simulink model "quadRotorController"  (R2016a)
settings: Solver=VariableStepAuto  StartTime=0.0  StopTime=100  RelTol=1e-3
libraries: simulink x1
settings Model: Creator=Nariman  LastModifiedBy=Nariman

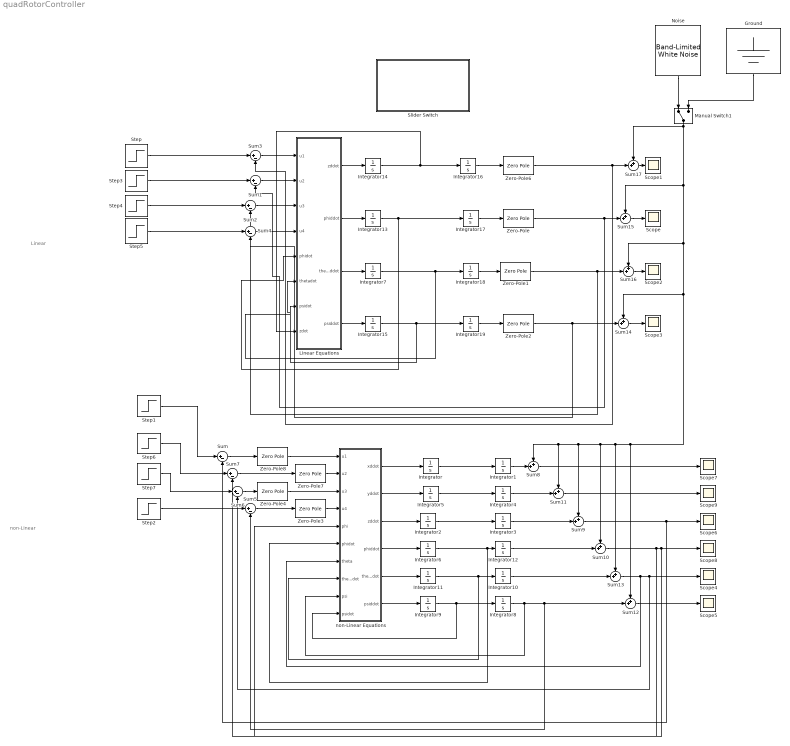
== system quadRotorController ==
  note: non-Linear
  note: Linear
  Ground : Ground
  Integrator{,1..19} (20 alike) : Integrator
  Linear Equations : MATLAB Function  TreatAsAtomicUnit=on
  Manual Switch1 : ManualSwitch
  Noise : simulink/Sources/Band-Limited White Noise  Cov=0.0000000001  Ts=0.1  seed=[23341]
  Scope{,1..9} (10 alike) : Scope
  Slider Switch : Subsystem  DialogController=hmiCreateDDGDialog  IsWebBlock=on  mask(MWDashboardBlock){webBlockId=d59a5245-7345-4851-88b2-e95f32656578, webBlockType=sliderswitch, ShowInLibBrowser=on, ShowInitialText=on, HMISrcModelName=model}
      mask prompts: webBlockId "WebBlock Id"; webBlockType "WebBlock Type"; HMISrcModelName "Source Model"
      mask Help: helpview([docroot '/mapfiles/simulink.map'], 'hmi_slider_switch')
      mask Display:
      | if strcmp(get_param(bdroot(gcb),'BlockDiagramType'), 'library')
      |     image([(matlabroot) '/toolbox/simulink/hmi/icons/SliderSwitch.png']);
      | end
  Step{,3..7} (6 alike) : Step  After=0.01  SampleTime=0
  Step1 : Step  After=90  SampleTime=0
  Step2 : Step  After=90  SampleTime=0
  Sum{,1..7} (8 alike) : Sum  Inputs=|+-
  Sum{8..17} (10 alike) : Sum  Inputs=++|
  Zero-Pole : ZeroPole  Zeros=[-0.949]  Poles=[-49]  Gain=[290]
  Zero-Pole1 : ZeroPole  Zeros=[-0.949]  Poles=[-49]  Gain=[100]
  Zero-Pole2 : ZeroPole  Zeros=[-0.3]  Poles=[-16.1]  Gain=[3.58]
  Zero-Pole3 : ZeroPole  Zeros=[-0.3]  Poles=[-16.1]  Gain=[3.58]
  Zero-Pole4 : ZeroPole  Zeros=[-0.949]  Poles=[-49]  Gain=[50]
  Zero-Pole6 : ZeroPole  Zeros=[-0.3]  Poles=[-16.1]  Gain=[90.58]
  Zero-Pole7 : ZeroPole  Zeros=[-0.949]  Poles=[-49]  Gain=[290]
  Zero-Pole8 : ZeroPole  Zeros=[-0.3]  Poles=[-16.1]  Gain=[90.58]
  non-Linear Equations : MATLAB Function  TreatAsAtomicUnit=on
  wires:
  non-Linear Equations/1(xddot) -> Integrator/1
  Integrator/1 -> Integrator1/1
  non-Linear Equations/2(yddot) -> Integrator5/1
  Integrator5/1 -> Integrator4/1
  non-Linear Equations/3(zddot) -> Integrator2/1
  Integrator2/1 -> Integrator3/1
  non-Linear Equations/4(phiddot) -> Integrator6/1
  Integrator6/1 -> non-Linear Equations/6(phidot), Integrator12/1
  non-Linear Equations/5(thetaddot) -> Integrator11/1
  Integrator11/1 -> Integrator10/1, non-Linear Equations/8(thetadot)
  non-Linear Equations/6(psiddot) -> Integrator9/1
  Integrator9/1 -> Integrator8/1, non-Linear Equations/10(psidot)
  Linear Equations/4(psiddot) -> Integrator15/1
  Linear Equations/3(thetaddot) -> Integrator7/1
  Linear Equations/2(phiddot) -> Integrator13/1
  Linear Equations/1(zddot) -> Integrator14/1
  Integrator15/1 -> Linear Equations/7(psidot), Integrator19/1
  Integrator7/1 -> Linear Equations/6(thetadot), Integrator18/1
  Integrator13/1 -> Integrator17/1, Linear Equations/5(phidot)
  Integrator14/1 -> Integrator16/1, Linear Equations/8(zdot)
  Integrator17/1 -> Zero-Pole/1
  Integrator18/1 -> Zero-Pole1/1
  Zero-Pole/1 -> Sum15/2, Sum1/2
  Sum3/1 -> Linear Equations/1(u1)
  Step/1 -> Sum3/1
  Sum1/1 -> Linear Equations/2(u2)
  Sum2/1 -> Linear Equations/3(u3)
  Sum4/1 -> Linear Equations/4(u4)
  Zero-Pole1/1 -> Sum16/2, Sum2/2
  Integrator19/1 -> Zero-Pole2/1
  Zero-Pole2/1 -> Sum14/2, Sum4/2
  Integrator16/1 -> Zero-Pole6/1
  Zero-Pole6/1 -> Sum17/2, Sum3/2
  Zero-Pole8/1 -> non-Linear Equations/1(u1)
  Sum/1 -> Zero-Pole8/1
  Sum7/1 -> Zero-Pole7/1
  Zero-Pole7/1 -> non-Linear Equations/2(u2)
  Sum6/1 -> Zero-Pole4/1
  Zero-Pole4/1 -> non-Linear Equations/3(u3)
  Zero-Pole3/1 -> non-Linear Equations/4(u4)
  Sum8/1 -> Scope7/1
  Integrator1/1 -> Sum8/2
  Integrator4/1 -> Sum11/2
  Sum11/1 -> Scope9/1
  Sum9/1 -> Sum/2, Scope6/1
  Integrator3/1 -> Sum9/2
  Integrator8/1 -> Sum12/2, Sum5/2, non-Linear Equations/9(psi)
  Integrator12/1 -> Sum10/2
  Sum10/1 -> non-Linear Equations/5(phi), Scope8/1, Sum7/2
  Integrator10/1 -> Sum13/2
  Sum13/1 -> Scope4/1, Sum6/2, non-Linear Equations/7(theta)
  Sum5/1 -> Zero-Pole3/1
  Step1/1 -> Sum/1
  Sum12/1 -> Scope5/1
  Noise/1 -> Manual Switch1/1
  Ground/1 -> Manual Switch1/2
  Sum14/1 -> Scope3/1
  Sum17/1 -> Scope1/1
  Sum16/1 -> Scope2/1
  Sum15/1 -> Scope/1
  Manual Switch1/1 -> Sum17/1, Sum15/1, Sum16/1, Sum14/1, Sum12/1, Sum13/1, Sum9/1, Sum11/1, Sum8/1, Sum10/1
  Step2/1 -> Sum5/1
  Step3/1 -> Sum1/1
  Step4/1 -> Sum2/1
  Step5/1 -> Sum4/1
  Step6/1 -> Sum7/1
  Step7/1 -> Sum6/1

== system quadRotorController/Slider Switch ==

== matlab function quadRotorController/Linear Equations ==
  data: u1 input; zddot output; u2 input; u3 input; u4 input; phidot input; thetadot input; psidot input; phiddot output; thetaddot output; psiddot output; zdot input
function [zddot,phiddot,thetaddot,psiddot] = fcn(u1,u2,u3,u4,phidot,thetadot,psidot,zdot)
ixx=0.0086;
iyy=0.0086;
izz=0.0176;
m=0.47;
zddot=zdot+u1/m;
phiddot=phidot+u2/ixx;
thetaddot=thetadot+u3/iyy;
psiddot=psidot+u4/izz;

== matlab function quadRotorController/non-Linear Equations ==
  data: u1 input; xddot output; u2 input; u3 input; u4 input; phi input; phidot input; theta input; thetadot input; psi input; psidot input; yddot output; zddot output; phiddot output; thetaddot output; psiddot output
function [xddot,yddot,zddot,phiddot,thetaddot,psiddot] = fcn(u1,u2,u3,u4,phi,phidot,theta,thetadot,psi,psidot)
g=9.8;
ixx=0.0086;
iyy=0.0086;
izz=0.0176;
m=0.47;
jr=3.74*10^(-5);
kf=3.13*10^(-5);
km=7.5*10^(-7);
l=0.44;
w1=sqrt(abs((1/(2*kf))*u1-(1/(4*kf*l))*u2));
w2=sqrt(abs((1/(4*kf))*u2-(1/(4*kf*l))*u3));
w3=sqrt(abs((1/(4*kf))*u2-(1/(2*kf*l))*u4));
w4=sqrt(abs((1/(2*kf))*u1-(1/(4*kf*l))*u2+(1/(4*kf*l))*u3+(1/(2*kf*l))*u4));
omegat=w1-w2+w3-w4;
xddot = (cos(psi)*sin(theta)*cos(phi)+sin(psi)*sin(phi))*u1/m;
yddot = (sin(psi)*sin(theta)*cos(phi)-sin(phi)*cos(psi))*u1/m;
zddot = (cos(theta)*cos(phi))*u1/m - g;
phiddot= (jr*thetadot*omegat/ixx)+((iyy-izz)/ixx)*psidot*thetadot+u2/ixx;
thetaddot= (jr*phidot*omegat/iyy)+((izz-ixx)/iyy)*psidot*phidot+u3/iyy;
psiddot= (ixx-iyy)*phidot*thetadot/izz + u4/izz;
